simulink model "quest4"  (R2015a)
settings: Solver=ode3  StartTime=0.0  StopTime=100  FixedStep=0.1  RelTol=1e-3
undefined symbols (not defined in the file or in its folder): lypo
libraries: simulink x2
settings Model: CovModelRefEnable=off  Creator=Subodh  LastModifiedBy=ecx
settings DataIOCC: SaveFormat=Dataset
settings HardwareCC: ProdBitPerPointer=64  ProdLargestAtomicFloat=Float  ProdIntDivRoundTo=Zero  ProdEndianess=LittleEndian  ProdHWDeviceType=Specified
settings GRTTargetCC: GeneratePreprocessorConditionals=Use local settings

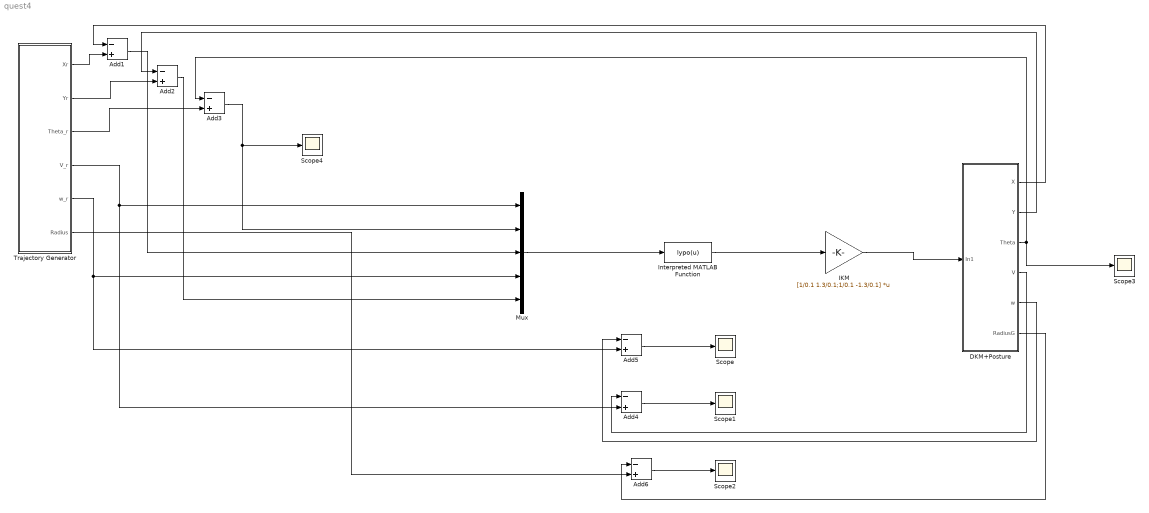
== system quest4 ==
  Add{1..6} (6 alike) : Sum  Inputs=-+
  DKM+Posture : Subsystem
  IKM : Gain  Gain=[1/0.1 1.3/0.1;1/0.1 -1.3/0.1]  Multiplication=Matrix(K*u)
  Interpreted MATLAB Function : MATLABFcn  MATLABFcn=lypo(u)  OutputDimensions=2
  Mux : Mux  Inputs=5
  Scope{,1..4} (5 alike) : Scope
      Scope settings: YMin=-0.07896  YMax=0.07617
      Scope1 settings: YMin=-2.70348  YMax=1.33134
      Scope2 settings: YMin=-0.52093  YMax=1.68833  SaveName=ScopeData2
      Scope3 settings: YMin=-0.07896  YMax=0.07617  SaveName=ScopeData3
      Scope4 settings: YMin=-0.07896  YMax=0.07617  SaveName=ScopeData4
  Trajectory Generator : Subsystem
  wires:
  Trajectory Generator/3(Theta_r) -> Add3/2
  DKM+Posture/1(X) -> Add1/1
  DKM+Posture/2(Y) -> Add2/1
  DKM+Posture/3(Theta) -> Add3/1, Scope3/1
  Trajectory Generator/4(V_r) -> Add4/2, Mux/1
  Trajectory Generator/5(w_r) -> Add5/2, Mux/4
  Add1/1 -> Mux/3
  Add2/1 -> Mux/5
  Mux/1 -> Interpreted MATLAB Function/1
  Interpreted MATLAB Function/1 -> IKM/1
  IKM/1 -> DKM+Posture/1(In1)
  Add5/1 -> Scope/1
  Add4/1 -> Scope1/1
  DKM+Posture/4(V) -> Add4/1
  DKM+Posture/5(w) -> Add5/1
  Trajectory Generator/6(Radius) -> Add6/2
  DKM+Posture/6(RadiusG) -> Add6/1
  Add6/1 -> Scope2/1
  Trajectory Generator/1(Xr) -> Add1/2
  Trajectory Generator/2(Yr) -> Add2/2
  Add3/1 -> Scope4/1, Mux/2

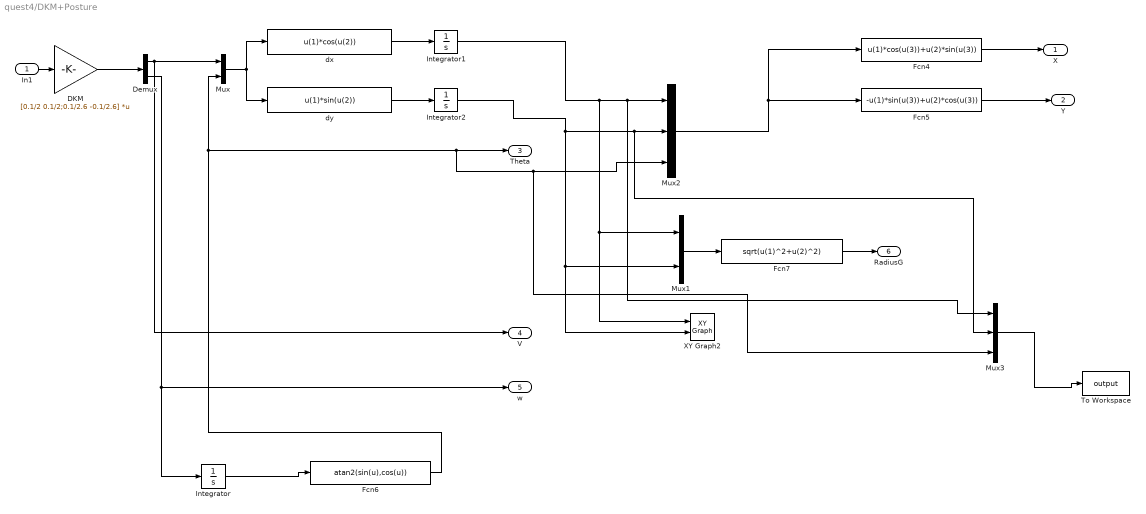
== system quest4/DKM+Posture ==
  In1 : Inport
  DKM : Gain  Gain=[0.1/2 0.1/2;0.1/2.6 -0.1/2.6]  Multiplication=Matrix(K*u)
  Demux : Demux  Outputs=2
  Fcn4 : Fcn  Expr=u(1)*cos(u(3))+u(2)*sin(u(3))
  Fcn5 : Fcn  Expr=-u(1)*sin(u(3))+u(2)*cos(u(3))
  Fcn6 : Fcn  Expr=atan2(sin(u),cos(u))
  Fcn7 : Fcn  Expr=sqrt(u(1)^2+u(2)^2)
  Integrator : Integrator  InitialCondition=pi
  Integrator1 : Integrator  InitialCondition=2.3
  Integrator2 : Integrator
  Mux : Mux  Inputs=2
  Mux1 : Mux  Inputs=2
  Mux2 : Mux  Inputs=3
  Mux3 : Mux  Inputs=3
  To Workspace : ToWorkspace  VariableName=output  SampleTime=-1
  XY Graph2 : simulink/Sinks/XY Graph  xmin=-2  xmax=2  ymin=-2  ymax=2  st=-1
  dx : Fcn  Expr=u(1)*cos(u(2))
  dy : Fcn  Expr=u(1)*sin(u(2))
  X : Outport
  Y : Outport  Port=2
  Theta : Outport  Port=3
  V : Outport  Port=4
  w : Outport  Port=5
  RadiusG : Outport  Port=6
  wires:
  Mux/1 -> dy/1, dx/1
  Demux/2 -> Integrator/1, w/1
  Demux/1 -> V/1, Mux/1
  dy/1 -> Integrator2/1
  Fcn6/1 -> Mux/2, Mux3/3, Mux2/3, Theta/1
  DKM/1 -> Demux/1
  In1/1 -> DKM/1
  dx/1 -> Integrator1/1
  Fcn4/1 -> X/1
  Fcn5/1 -> Y/1
  Integrator2/1 -> Mux1/2, XY Graph2/2, Mux3/2, Mux2/2
  Mux2/1 -> Fcn4/1, Fcn5/1
  Integrator/1 -> Fcn6/1
  Mux1/1 -> Fcn7/1
  Integrator1/1 -> XY Graph2/1, Mux1/1, Mux3/1, Mux2/1
  Fcn7/1 -> RadiusG/1
  Mux3/1 -> To Workspace/1

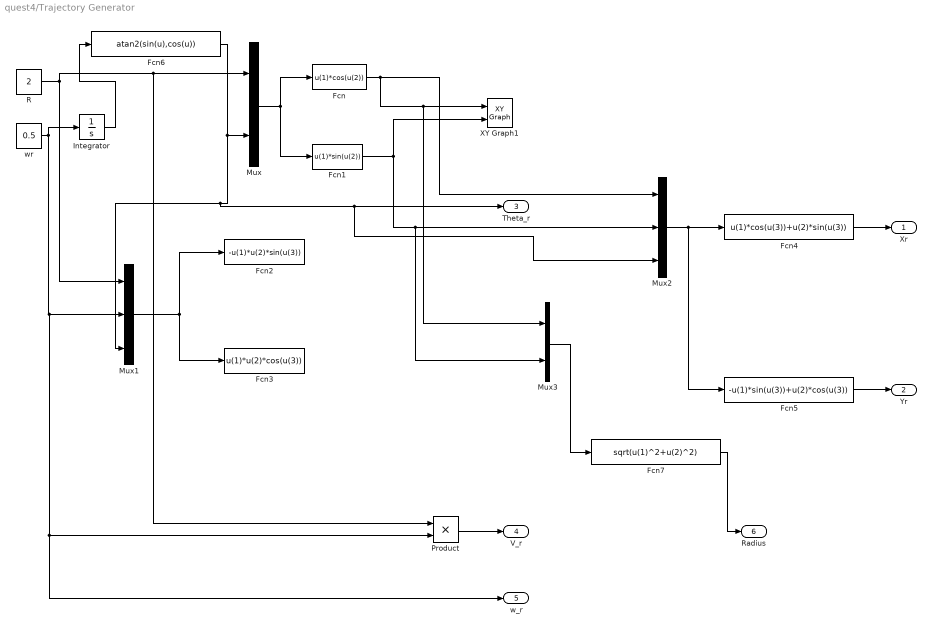
== system quest4/Trajectory Generator ==
  Fcn : Fcn  Expr=u(1)*cos(u(2))
  Fcn1 : Fcn  Expr=u(1)*sin(u(2))
  Fcn2 : Fcn  Expr=-u(1)*u(2)*sin(u(3))
  Fcn3 : Fcn  Expr=u(1)*u(2)*cos(u(3))
  Fcn4 : Fcn  Expr=u(1)*cos(u(3))+u(2)*sin(u(3))
  Fcn5 : Fcn  Expr=-u(1)*sin(u(3))+u(2)*cos(u(3))
  Fcn6 : Fcn  Expr=atan2(sin(u),cos(u))
  Fcn7 : Fcn  Expr=sqrt(u(1)^2+u(2)^2)
  Integrator : Integrator
  Mux : Mux  Inputs=2
  Mux1 : Mux  Inputs=3
  Mux2 : Mux  Inputs=3
  Mux3 : Mux  Inputs=2
  Product : Product
  R : Constant  Value=2
  XY Graph1 : simulink/Sinks/XY Graph  xmin=-2  xmax=2  ymin=-2  ymax=2  st=-1
  wr : Constant  Value=0.5
  Xr : Outport
  Yr : Outport  Port=2
  Theta_r : Outport  Port=3
  V_r : Outport  Port=4
  w_r : Outport  Port=5
  Radius : Outport  Port=6
  wires:
  Fcn/1 -> Mux3/1, XY Graph1/1, Mux2/1
  Mux1/1 -> Fcn2/1, Fcn3/1
  Fcn1/1 -> XY Graph1/2, Mux3/2, Mux2/2
  Mux/1 -> Fcn/1, Fcn1/1
  R/1 -> Mux1/1, Product/1, Mux/1
  wr/1 -> Integrator/1, w_r/1, Product/2, Mux1/2
  Fcn6/1 -> Mux2/3, Theta_r/1, Mux1/3, Mux/2
  Product/1 -> V_r/1
  Mux2/1 -> Fcn5/1, Fcn4/1
  Fcn4/1 -> Xr/1
  Fcn5/1 -> Yr/1
  Integrator/1 -> Fcn6/1
  Mux3/1 -> Fcn7/1
  Fcn7/1 -> Radius/1
